simulink model "testConnect"  (R2024b)
settings: Solver=VariableStepAuto  StartTime=0.0  StopTime=10.0  RelTol=1e-3
settings Model: Creator=grouleau  LastModifiedBy=grouleau

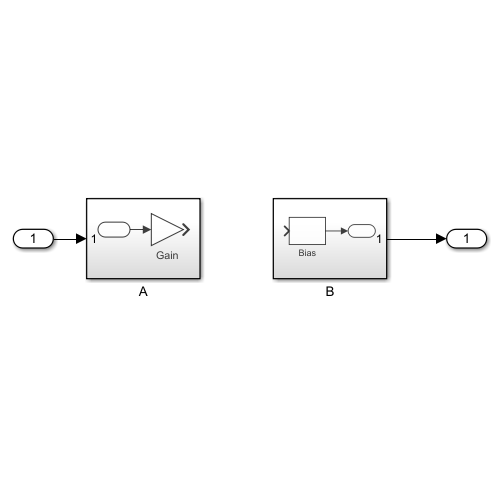
[thumbnail: Simulink's stored preview of the top-level diagram]
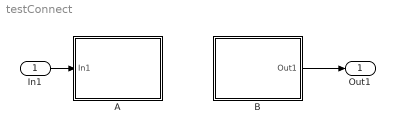
== system testConnect ==
  In1 : Inport
  A : Subsystem
  B : Subsystem
  Out1 : Outport
  wires:
  In1/1 -> A/1(In1)
  B/1(Out1) -> Out1/1

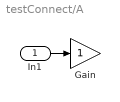
== system testConnect/A ==
  In1 : Inport
  Gain : Gain
  wires:
  In1/1 -> Gain/1

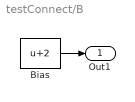
== system testConnect/B ==
  Bias : Bias  Bias=2  SaturateOnIntegerOverflow=off
  Out1 : Outport
  wires:
  Bias/1 -> Out1/1
